simulink model "sampleModel119"  (R2021b)
settings: Solver=VariableStepAuto  StartTime=0.0  StopTime=10.0  RelTol=1e-3
undefined symbols (not defined in the file or in its folder): DiscIntNeverNeededParam, Newton, Raphson
libraries: simulink x14, slpidlib x1
settings Model: Creator=user  LastModifiedBy=user

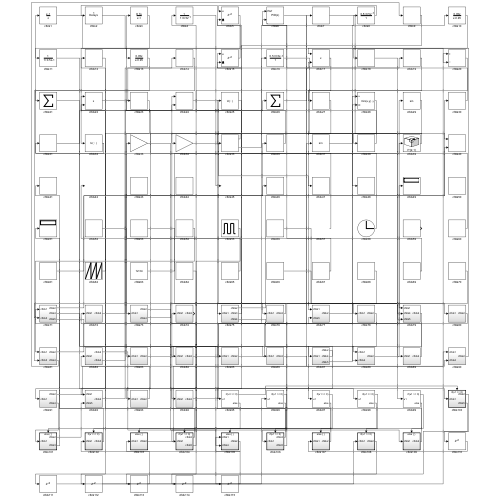
[thumbnail: Simulink's stored preview of the top-level diagram]
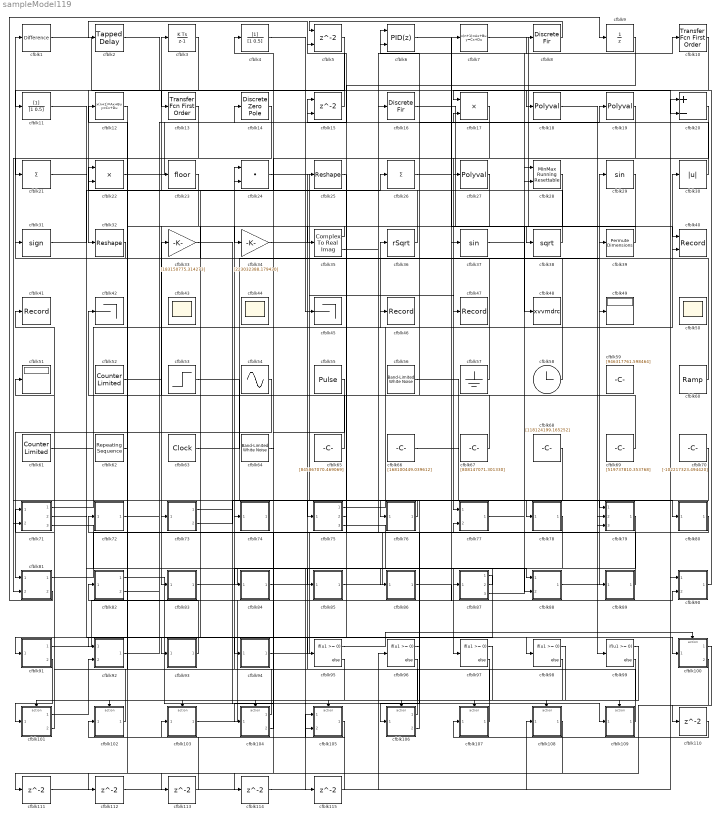
== system sampleModel119 ==
  cfblk1 : simulink/Discrete/Difference  ICPrevInput=0.0  OutMin=[]  OutMax=[]  OutDataTypeStr=Inherit: Inherit via back propagation  OutDataType=fixdt(1, 16)  OutScaling=2^-10  DoSatur=off
  cfblk10 : simulink/Discrete/Transfer Fcn First Order  PoleZ=0.95  ICPrevOutput=0.0  DoSatur=off
  cfblk100 : Subsystem  TreatAsAtomicUnit=on
  cfblk101 : Subsystem  TreatAsAtomicUnit=on
  cfblk102 : Subsystem  TreatAsAtomicUnit=on
  cfblk103 : Subsystem  TreatAsAtomicUnit=on
  cfblk104 : Subsystem  TreatAsAtomicUnit=on
  cfblk105 : Subsystem  TreatAsAtomicUnit=on
  cfblk106 : Subsystem  TreatAsAtomicUnit=on
  cfblk107 : Subsystem  TreatAsAtomicUnit=on
  cfblk108 : Subsystem  TreatAsAtomicUnit=on
  cfblk109 : Subsystem  TreatAsAtomicUnit=on
  cfblk11 : DiscreteFilter  SampleTime=1
  cfblk{110..115} (6 alike) : Delay  SampleTime=1
  cfblk12 : DiscreteStateSpace
  cfblk13 : simulink/Discrete/Transfer Fcn First Order  PoleZ=0.95  ICPrevOutput=0.0  DoSatur=off
  cfblk14 : DiscreteZeroPole  Poles=[0 0.5]  Gain=1
  cfblk15 : Delay  ShowEnablePort=on  SampleTime=1
      settings: InputPortMap=u0,e6
  cfblk16 : DiscreteFir  SampleTime=1
  cfblk17 : Product
  cfblk18 : Polyval  Coefs=[ +2.081618890e-019, -1.441693666e-014, +4.719686976e-010, -8.536869453e-006, +1.621573104e-001, -8.087801117e+001 ]
  cfblk19 : Polyval  Coefs=[ +2.081618890e-019, -1.441693666e-014, +4.719686976e-010, -8.536869453e-006, +1.621573104e-001, -8.087801117e+001 ]
  cfblk2 : simulink/Discrete/Tapped Delay  vinit=0.0  samptime=-1  NumDelays=1  DelayOrder=Oldest  includeCurrent=off
  cfblk20 : Sum  Inputs=+-
  cfblk21 : Sum  Inputs=+
  cfblk22 : Product  Inputs=**
  cfblk23 : Rounding
  cfblk24 : DotProduct  InputSameDT=on  OutDataTypeStr=Inherit: Inherit via internal rule
  cfblk25 : Reshape
  cfblk26 : Sum  Inputs=+
  cfblk27 : Polyval  Coefs=[ +2.081618890e-019, -1.441693666e-014, +4.719686976e-010, -8.536869453e-006, +1.621573104e-001, -8.087801117e+001 ]
  cfblk28 : simulink/Math Operations/MinMax Running Resettable  Function=min  vinit=0.0
  cfblk29 : Trigonometry
  cfblk3 : DiscreteIntegrator  ICPrevOutput=DiscIntNeverNeededParam  ICPrevScaledInput=DiscIntNeverNeededParam
  cfblk30 : Abs
  cfblk31 : Signum
  cfblk32 : Reshape
  cfblk33 : Gain  Gain=[183150775.314273]
  cfblk34 : Gain  Gain=[223032388.179430]
  cfblk35 : ComplexToRealImag
  cfblk36 : Sqrt  Operator=rSqrt  AlgorithmType=Newton-Raphson  SaturateOnIntegerOverflow=on
  cfblk37 : Trigonometry
  cfblk38 : Sqrt  SaturateOnIntegerOverflow=on
  cfblk39 : PermuteDimensions
  cfblk4 : DiscreteFilter  SampleTime=1
  cfblk40 : Record  FileSettingsInternal="{\"entries\":[{\"content\":{\"excelSettings\":{\"content\":{},\"type\":\"Streamout.ExcelSettings\"}},\"type\":\"Streamout.FileSettingStorage\",\"uuid\":\"4b90652c-f2d3-47f2-a44e-bcf3a3fec26d\"}],\"packageUris\":[\"http://schema.mathworks.com/mf0/streamout_blocks/R2020a\"],\"version\":\"1.0\"}"  Layout=[1 1]  SignalsInternal="{\"entries\":[{\"content\":{\"signals\":[{\"content\":{\"blockPath\":[\"sampleModel119/cfblk40\"],\"channel\":[],\"dimensions\":[1],\"domain\":\"sampleModel119/cfblk40\",\"lineColor\":\"#a2142f\",\"plots\":[1],\"port\":1,\"sid\":[\"\"],\"signalID\":4151,\"signalName\":\"cfblk6\"},\"type\":\"RecordBlkView.Signal\",\"uuid\":\"d5e0444b-39c8-4732-8124-8d2ee03c9154\"},{\"content\":{\"blockPath\":[\"sampleModel119/cfblk40\"],\"channel\":[],\"dimensions\":[1],\"domain\":\"sampleModel119/cfblk40\",\"lineColor\":\"#139fff\",\"plots\":[1],\"port\":2,\"sid\":[\"\"],\"signalID\":4155,\"signalName\":\"cfblk61\"},\"type\":\"RecordBlkView.Signal\",\"uuid\":\"776bc78c-e7e2-49e1-a7fd-18f1511b43d9\"}]},\"type\":\"RecordBlkView.InputSignals\",\"uuid\":\"2fea9de3-cc0b-4d57-9cd3-248ab124d388\"}],\"packageUris\":[\"http://schema.mathworks.com/mf0/streamout_blocks/R2020a\"],\"version\":\"1.0\"}"  VisualizationBindings="{\"xyplotplugin\":{\"info\":[{\"series\":[{\"bindingParametersList\":[{\"parameter\":\"X-Axis\",\"signalID\":4151,\"signalName\":\"cfblk6\"},{\"parameter\":\"Y-Axis\",\"signalID\":4155,\"signalName\":\"cfblk61\"}],\"seriesID\":3220}],\"subplotID\":1}]}}"  CompatibilityTag=XY
  cfblk41 : Record  FileSettingsInternal="{\"entries\":[{\"content\":{\"excelSettings\":{\"content\":{},\"type\":\"Streamout.ExcelSettings\"}},\"type\":\"Streamout.FileSettingStorage\",\"uuid\":\"8c36c4d4-0469-459e-8325-57697a053134\"}],\"packageUris\":[\"http://schema.mathworks.com/mf0/streamout_blocks/R2020a\"],\"version\":\"1.0\"}"  SignalsInternal="{\"entries\":[{\"content\":{\"signals\":[{\"content\":{\"blockPath\":[\"sampleModel119/cfblk41\"],\"channel\":[],\"dimensions\":[1],\"domain\":\"sampleModel119/cfblk41\",\"lineColor\":\"#fe330a\",\"plots\":[1],\"port\":1,\"sid\":[\"\"],\"signalID\":4159,\"signalName\":\"cfblk104:1\"},\"type\":\"RecordBlkView.Signal\",\"uuid\":\"6d2d44fb-15cd-4da0-8e52-60f91c5e197b\"}]},\"type\":\"RecordBlkView.InputSignals\",\"uuid\":\"76cdbd26-62aa-4d26-a689-d7fa7566e8ef\"}],\"packageUris\":[\"http://schema.mathworks.com/mf0/streamout_blocks/R2020a\"],\"version\":\"1.0\"}"  VisualizationBindings="{\"sparklinesplugin\":{\"info\":[{\"bindingParametersList\":[],\"subplotID\":1}]}}"
  cfblk42 : Terminator
  cfblk43 : Scope
      settings: Floating=on
  cfblk44 : Scope
      settings: Floating=on
  cfblk45 : Terminator
  cfblk46 : Record  FileSettingsInternal="{\"entries\":[{\"content\":{\"excelSettings\":{\"content\":{},\"type\":\"Streamout.ExcelSettings\"}},\"type\":\"Streamout.FileSettingStorage\",\"uuid\":\"35d2fa41-f68c-4e08-ac86-24c0cc6052f6\"}],\"packageUris\":[\"http://schema.mathworks.com/mf0/streamout_blocks/R2020a\"],\"version\":\"1.0\"}"  SignalsInternal="{\"entries\":[{\"content\":{\"signals\":[{\"content\":{\"blockPath\":[\"sampleModel119/cfblk46\"],\"channel\":[],\"dimensions\":[1],\"domain\":\"sampleModel119/cfblk46\",\"lineColor\":\"#22b573\",\"plots\":[1],\"port\":1,\"sid\":[\"\"],\"signalID\":4163,\"signalName\":\"cfblk72\"},\"type\":\"RecordBlkView.Signal\",\"uuid\":\"6c816a1f-c12f-4d80-813e-4e8bf75e3cfa\"}]},\"type\":\"RecordBlkView.InputSignals\",\"uuid\":\"aab32150-6d44-4daa-b8cf-e47eaa1a11c6\"}],\"packageUris\":[\"http://schema.mathworks.com/mf0/streamout_blocks/R2020a\"],\"version\":\"1.0\"}"  VisualizationBindings="{\"sparklinesplugin\":{\"info\":[{\"bindingParametersList\":[],\"subplotID\":1}]}}"
  cfblk47 : Record  FileSettingsInternal="{\"entries\":[{\"content\":{\"excelSettings\":{\"content\":{},\"type\":\"Streamout.ExcelSettings\"}},\"type\":\"Streamout.FileSettingStorage\",\"uuid\":\"1cc15422-dbef-4f88-bbe8-034119ca05b7\"}],\"packageUris\":[\"http://schema.mathworks.com/mf0/streamout_blocks/R2020a\"],\"version\":\"1.0\"}"  SignalsInternal="{\"entries\":[{\"content\":{\"signals\":[{\"content\":{\"blockPath\":[\"sampleModel119/cfblk47\"],\"channel\":[],\"dimensions\":[1,1],\"domain\":\"sampleModel119/cfblk47\",\"lineColor\":\"#0072bd\",\"plots\":[1],\"port\":1,\"sid\":[\"\"],\"signalID\":4167,\"signalName\":\"cfblk34\"},\"type\":\"RecordBlkView.Signal\",\"uuid\":\"1ed8d035-bae1-4148-97b8-32f6098d1f51\"}]},\"type\":\"RecordBlkView.InputSignals\",\"uuid\":\"92e54281-6170-43a9-afc8-92f9430844b9\"}],\"packageUris\":[\"http://schema.mathworks.com/mf0/streamout_blocks/R2020a\"],\"version\":\"1.0\"}"  VisualizationBindings="{\"sparklinesplugin\":{\"info\":[{\"bindingParametersList\":[],\"subplotID\":1}]}}"
  cfblk48 : ToWorkspace  VariableName=xvvmdrc  SaveFormat=Timeseries  SampleTime=-1
  cfblk49 : Display
  cfblk5 : Delay  ShowEnablePort=on  SampleTime=1
      settings: InputPortMap=u0,e6
  cfblk50 : Scope
      settings: Floating=on
  cfblk51 : Display
  cfblk52 : simulink/Sources/Counter Limited  uplimit=[61.000000]  tsamp=-1
  cfblk53 : Step  Time=[34.000000]  Before=[46179549.003824]  After=[835001809.897906]  SampleTime=0
  cfblk54 : Sin  Amplitude=[-89702734.800295]  Bias=[573127760.762597]  SampleTime=0
  cfblk55 : DiscretePulseGenerator  PulseType=Time based  Amplitude=[-241727286.164151]  Period=[40925784.883433]  PulseWidth=5  PhaseDelay=[9.000000]
  cfblk56 : simulink/Sources/Band-Limited White Noise  Cov=[2484773712.290704]  Ts=0.1  seed=[484627539.000000]
  cfblk57 : Ground
  cfblk58 : Clock
  cfblk59 : Constant  Value=[946317761.598464]  SampleTime=1
  cfblk6 : slpidlib/PID Controller (2DOF)  Controller=PID  Form=Parallel  TimeDomain=Discrete-time  UseExternalTs=off  SampleTime=1  IntegratorMethod=Forward Euler  FilterMethod=Forward Euler  ControllerParametersSource=internal  P=1  I=1  D=0  UseFilter=on  N=100  b=1  c=1  TunerSelectOption=Transfer Function Based (PID Tuner App)  InitialConditionSource=internal  InitialConditionForIntegrator=0  InitialConditionForFilter=0  DifferentiatorICPrevScaledInput=0  ExternalReset=none  TrackingMode=off  Kt=1  LimitOutput=off  SatLimitsSource=internal  UpperSaturationLimit=inf  LowerSaturationLimit=-inf  LinearizeAsGain=off  AntiWindupMode=none  Kb=1  POutMin=[]  POutMax=[]  IOutMin=[]  IOutMax=[]  DOutMin=[]  DOutMax=[]  NOutMin=[]  NOutMax=[]  bOutMin=[]  bOutMax=[]  cOutMin=[]  cOutMax=[]  SumOutMin=[]  SumOutMax=[]  SaturationOutMin=[]  SaturationOutMax=[]  PParamMin=[]  PParamMax=[]  IParamMin=[]  IParamMax=[]  DParamMin=[]  DParamMax=[]  NParamMin=[]  NParamMax=[]  bParamMin=[]  bParamMax=[]  cParamMin=[]  cParamMax=[]  KbParamMin=[]  KbParamMax=[]  KtParamMin=[]  KtParamMax=[]  KbOutMin=[]  KbOutMax=[]  KtOutMin=[]  KtOutMax=[]  IntegratorOutMin=[]  IntegratorOutMax=[]  FilterOutMin=[]  FilterOutMax=[]  SumI1OutMin=[]  SumI1OutMax=[]  SumI2OutMin=[]  SumI2OutMax=[]  SumI3OutMin=[]  SumI3OutMax=[]  SumI4OutMin=[]  SumI4OutMax=[]  SumDOutMin=[]  SumDOutMax=[]  Sum1OutMin=[]  Sum1OutMax=[]  Sum2OutMin=[]  Sum2OutMax=[]  Sum3OutMin=[]  Sum3OutMax=[]  DifferentiatorOutMin=[]  DifferentiatorOutMax=[]  FilterDiffOutCoefMin=[]  FilterDiffOutCoefMax=[]  ReciprocalOutMin=[]  ReciprocalOutMax=[]  SumDenOutMin=[]  SumDenOutMax=[]  SumNumOutMin=[]  SumNumOutMax=[]  DivideOutMin=[]  DivideOutMax=[]  UdiffTsProdOutMin=[]  UdiffTsProdOutMax=[]  NTsProdOutMin=[]  NTsProdOutMax=[]  UintegralTsProdOutMin=[]  UintegralTsProdOutMax=[]  UngainTsProdOutMin=[]  UngainTsProdOutMax=[]  IntegratorContinuousStateAttributes=''  IntegratorStateMustResolveToSignalObject=off  IntegratorRTWStateStorageClass=Auto  FilterContinuousStateAttributes=''  FilterStateMustResolveToSignalObject=off  FilterRTWStateStorageClass=Auto  ParallelPVariant=InternalParameters  IdealPVariant=Disabled  IVariant=InternalParameters  DVariant=InternalParameters  bVariant=InternalParameters  cVariant=InternalParameters  IntegratorVariant=Discrete  SatVariant=Disabled  AWVariant=Passthrough  PCopyVariant=Disabled  TRVariant=Disabled  FdbkBlocksVariant=Forward  IdealPFdbkVariant=Disabled  SatFdbkVariant=Disabled  DerivativeFilterVariant=ForwardEulerFilter  NVariant=InternalParameters  NCopyVariant=Disabled  FilterICVariant=InternalICsFilter  IntegratorICVariant=InternalICs  ExternalResetVariant=Disabled  TRSumVariant=Passthrough  SumFdbkVariant=Disabled  SumVariant=Sum_PID  TsampFilterVariant=InternalTs  TsampNgainVariant=Passthrough  TsampIntegralVariant=Passthrough  ExternalSaturationOutDataTypeStr=Inherit: Same as second input
      settings: SourceProductBaseCode=SL
  cfblk60 : simulink/Sources/Ramp  slope=[5825.161716]  start=[33.046930]  InitialOutput=[-744615.276232]
  cfblk61 : simulink/Sources/Counter Limited  uplimit=[442.000000]  tsamp=-1
  cfblk62 : simulink/Sources/Repeating Sequence  rep_seq_t=[0 2]  rep_seq_y=[-993841258.890816, 268026566.571388]
  cfblk63 : DigitalClock
  cfblk64 : simulink/Sources/Band-Limited White Noise  Cov=[6507311425.437892]  Ts=0.1  seed=[1699256714.000000]
  cfblk65 : Constant  Value=[845867070.469069]  SampleTime=1
  cfblk66 : Constant  Value=[168100449.039612]  SampleTime=1
  cfblk67 : Constant  Value=[808147071.301330]  SampleTime=1
  cfblk68 : Constant  Value=[118124199.165252]  SampleTime=1
  cfblk69 : Constant  Value=[519737810.353768]  SampleTime=1
  cfblk7 : DiscreteStateSpace
  cfblk70 : Constant  Value=[-102217323.494420]  SampleTime=1
  cfblk71 : Subsystem
  cfblk72 : Subsystem
  cfblk73 : Subsystem
  cfblk74 : Subsystem
  cfblk75 : Subsystem
  cfblk76 : Subsystem
  cfblk77 : Subsystem
  cfblk78 : Subsystem
  cfblk79 : Subsystem
  cfblk8 : DiscreteFir  SampleTime=1
  cfblk80 : Subsystem
  cfblk81 : Subsystem
  cfblk82 : Subsystem
  cfblk83 : Subsystem
  cfblk84 : Subsystem
  cfblk85 : Subsystem
  cfblk86 : Subsystem
  cfblk87 : Subsystem
  cfblk88 : Subsystem
  cfblk89 : Subsystem
  cfblk9 : UnitDelay  HasFrameUpgradeWarning=on
  cfblk90 : Subsystem
  cfblk91 : Subsystem
  cfblk92 : Subsystem
  cfblk93 : Subsystem
  cfblk94 : Subsystem
  cfblk{95..99} (5 alike) : If  IfExpression=u1 >= 0  SampleTime=1
  wires:
  cfblk93/1(cfblk2) -> cfblk82/1(cfblk1)
  cfblk3/1 -> cfblk32/1
  cfblk63/1 -> cfblk29/1
  cfblk81/1(cfblk2) -> cfblk39/1
  cfblk106/1(cfblk2) -> cfblk24/1
  cfblk105/1(cfblk2) -> cfblk102/1(cfblk1)
  cfblk19/1 -> cfblk77/1(cfblk1)
  cfblk78/1(cfblk2) -> cfblk97/1
  cfblk38/1 -> cfblk3/1
  cfblk53/1 -> cfblk76/1(cfblk1)
  cfblk24/1 -> cfblk78/1(cfblk1)
  cfblk1/1 -> cfblk13/1
  cfblk32/1 -> cfblk1/1
  cfblk91/1(cfblk2) -> cfblk37/1
  cfblk80/1(cfblk2) -> cfblk77/2(cfblk5)
  cfblk83/1(cfblk2) -> cfblk87/1(cfblk1)
  cfblk109/1(cfblk2) -> cfblk25/1
  cfblk29/1 -> cfblk38/1
  cfblk76/1(cfblk2) -> cfblk75/1(cfblk1)
  cfblk107/1(cfblk2) -> cfblk12/1
  cfblk82/1(cfblk2) -> cfblk109/1(cfblk1)
  cfblk75/1(cfblk2) -> cfblk30/1
  cfblk87/1(cfblk2) -> cfblk91/1(cfblk1)
  cfblk16/1 -> cfblk48/1
  cfblk62/1 -> cfblk22/1
  cfblk66/1 -> cfblk80/1(cfblk1)
  cfblk87/2(cfblk4) -> cfblk84/1(cfblk1)
  cfblk106/2(cfblk5) -> cfblk72/1(cfblk1)
  cfblk90/1(cfblk2) -> cfblk17/1
  cfblk35/1 -> cfblk34/1
  cfblk71/1(cfblk2) -> cfblk36/1
  cfblk4/1 -> cfblk45/1
  cfblk54/1 -> cfblk81/1(cfblk1)
  cfblk103/1(cfblk2) -> cfblk20/1
  cfblk15/1 -> cfblk2/1
  cfblk88/1(cfblk2) -> cfblk49/1
  cfblk9/1 -> cfblk15/1
  cfblk22/1 -> cfblk17/2
  cfblk60/1 -> cfblk31/1
  cfblk84/1(cfblk2) -> cfblk7/1
  cfblk34/1 -> cfblk47/1
  cfblk52/1 -> cfblk83/1(cfblk1)
  cfblk7/1 -> cfblk89/1(cfblk1)
  cfblk94/1(cfblk2) -> cfblk16/1
  cfblk23/1 -> cfblk73/1(cfblk1)
  cfblk102/1(cfblk2) -> cfblk71/1(cfblk1)
  cfblk2/1 -> cfblk20/2
  cfblk6/1 -> cfblk40/1
  cfblk68/1 -> cfblk71/2(cfblk3)
  cfblk87/3(cfblk5) -> cfblk28/1
  cfblk64/1 -> cfblk94/1(cfblk1)
  cfblk14/1 -> cfblk21/1
  cfblk30/1 -> cfblk6/1
  cfblk67/1 -> cfblk33/1
  cfblk70/1 -> cfblk106/1(cfblk1)
  cfblk104/1(cfblk2) -> cfblk41/1
  cfblk55/1 -> cfblk104/1(cfblk1)
  cfblk58/1 -> cfblk23/1
  cfblk104/2(cfblk5) -> cfblk74/1(cfblk1)
  cfblk85/1(cfblk2) -> cfblk28/2
  cfblk65/1 -> cfblk42/1
  cfblk39/1 -> cfblk35/1
  cfblk35/2 -> cfblk8/1
  cfblk20/1 -> cfblk27/1
  cfblk31/1 -> cfblk24/2
  cfblk73/1(cfblk2) -> cfblk100/1(cfblk1)
  cfblk8/1 -> cfblk5/1
  cfblk91/2(cfblk4) -> cfblk101/1(cfblk1)
  cfblk57/1 -> cfblk5/2
  cfblk72/1(cfblk2) -> cfblk46/1
  cfblk82/2(cfblk4) -> cfblk14/1
  cfblk71/2(cfblk4) -> cfblk85/1(cfblk1)
  cfblk37/1 -> cfblk10/1
  cfblk75/2(cfblk3) -> cfblk22/2
  cfblk56/1 -> cfblk99/1
  cfblk13/1 -> cfblk81/2(cfblk3)
  cfblk33/1 -> cfblk105/2(cfblk4)
  cfblk36/1 -> cfblk4/1
  cfblk12/1 -> cfblk92/1(cfblk1)
  cfblk25/1 -> cfblk95/1
  cfblk10/1 -> cfblk18/1
  cfblk21/1 -> cfblk86/1(cfblk1)
  cfblk75/3(cfblk4) -> cfblk88/1(cfblk1)
  cfblk73/2(cfblk4) -> cfblk79/1(cfblk1)
  cfblk61/1 -> cfblk40/2
  cfblk5/1 -> cfblk11/1
  cfblk28/1 -> cfblk93/1(cfblk1)
  cfblk89/1(cfblk2) -> cfblk15/2
  cfblk81/2(cfblk4) -> cfblk9/1
  cfblk11/1 -> cfblk98/1
  cfblk77/1(cfblk2) -> cfblk79/2(cfblk4)
  cfblk79/1(cfblk2) -> cfblk88/2(cfblk4)
  cfblk101/1(cfblk2) -> cfblk92/2(cfblk5)
  cfblk101/2(cfblk3) -> cfblk51/1
  cfblk18/1 -> cfblk79/3(cfblk5)
  cfblk69/1 -> cfblk6/2
  cfblk26/1 -> cfblk19/1
  cfblk86/1(cfblk2) -> cfblk90/2(cfblk4)
  cfblk92/1(cfblk2) -> cfblk26/1
  cfblk95/1 -> cfblk100/Action
  cfblk95/2 -> cfblk101/Action
  cfblk96/1 -> cfblk102/Action
  cfblk96/2 -> cfblk103/Action
  cfblk97/1 -> cfblk104/Action
  cfblk97/2 -> cfblk105/Action
  cfblk98/1 -> cfblk106/Action
  cfblk98/2 -> cfblk107/Action
  cfblk99/1 -> cfblk108/Action
  cfblk99/2 -> cfblk109/Action
  cfblk100/1(cfblk2) -> cfblk110/1
  cfblk110/1 -> cfblk107/1(cfblk1)
  cfblk100/2(cfblk5) -> cfblk111/1
  cfblk111/1 -> cfblk96/1
  cfblk27/1 -> cfblk112/1
  cfblk112/1 -> cfblk108/1(cfblk1)
  cfblk108/1(cfblk2) -> cfblk113/1
  cfblk113/1 -> cfblk103/1(cfblk1)
  cfblk17/1 -> cfblk114/1
  cfblk114/1 -> cfblk90/1(cfblk1)
  cfblk71/3(cfblk5) -> cfblk115/1
  cfblk115/1 -> cfblk105/1(cfblk1)

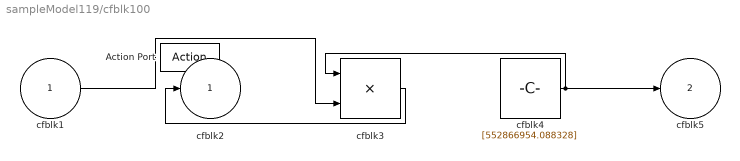
== system sampleModel119/cfblk100 ==
  cfblk1 : Inport
  Action Port : ActionPort  ActionPortLabel=if(u1 >= 0)
  cfblk3 : Product  Inputs=**
  cfblk4 : Constant  Value=[552866954.088328]  SampleTime=1
  cfblk2 : Outport
  cfblk5 : Outport  Port=2
  wires:
  cfblk4/1 -> cfblk3/1, cfblk5/1
  cfblk3/1 -> cfblk2/1
  cfblk1/1 -> cfblk3/2

== system sampleModel119/cfblk101 ==
  cfblk1 : Inport
  Action Port : ActionPort  ActionPortLabel=else
  cfblk2 : Outport
  cfblk3 : Outport  Port=2
  wires:
  cfblk1/1 -> cfblk3/1, cfblk2/1

== system sampleModel119/cfblk102 ==
  cfblk1 : Inport
  Action Port : ActionPort  ActionPortLabel=if(u1 >= 0)
  cfblk3 : simulink/Discrete/Transfer Fcn Real Zero  ZeroZ=0.75  ICPrevInput=0.0  DoSatur=off
      settings: SourceProductBaseCode=SL
  cfblk2 : Outport
  wires:
  cfblk3/1 -> cfblk2/1
  cfblk1/1 -> cfblk3/1

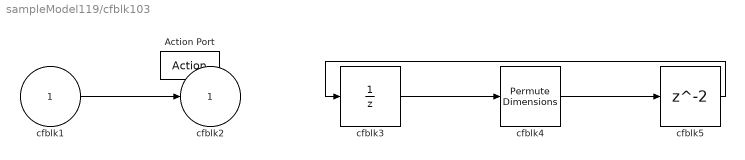
== system sampleModel119/cfblk103 ==
  cfblk1 : Inport
  Action Port : ActionPort  ActionPortLabel=else
  cfblk3 : UnitDelay  SampleTime=-1  HasFrameUpgradeWarning=on
  cfblk4 : PermuteDimensions
  cfblk5 : Delay
  cfblk2 : Outport
  wires:
  cfblk1/1 -> cfblk2/1
  cfblk3/1 -> cfblk4/1
  cfblk4/1 -> cfblk5/1
  cfblk5/1 -> cfblk3/1

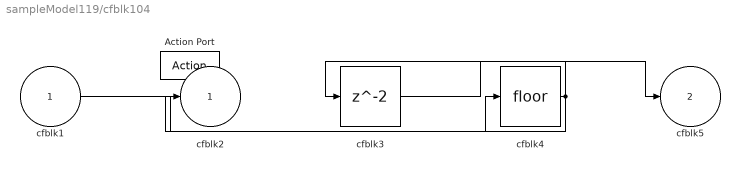
== system sampleModel119/cfblk104 ==
  cfblk1 : Inport
  Action Port : ActionPort  ActionPortLabel=if(u1 >= 0)
  cfblk3 : Delay
  cfblk4 : Rounding
  cfblk2 : Outport
  cfblk5 : Outport  Port=2
  wires:
  cfblk1/1 -> cfblk4/1
  cfblk4/1 -> cfblk3/1, cfblk2/1
  cfblk3/1 -> cfblk5/1

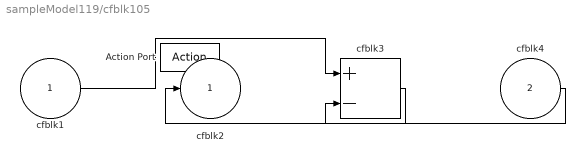
== system sampleModel119/cfblk105 ==
  cfblk1 : Inport
  cfblk4 : Inport  Port=2
  Action Port : ActionPort  ActionPortLabel=else
  cfblk3 : Sum  Inputs=+-
  cfblk2 : Outport
  wires:
  cfblk3/1 -> cfblk2/1
  cfblk1/1 -> cfblk3/1
  cfblk4/1 -> cfblk3/2

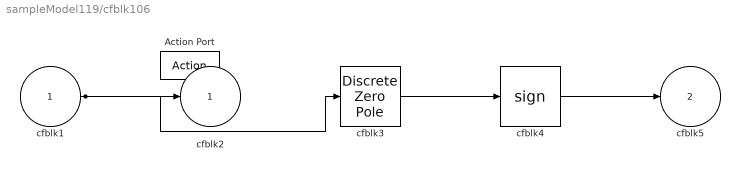
== system sampleModel119/cfblk106 ==
  cfblk1 : Inport
  Action Port : ActionPort  ActionPortLabel=if(u1 >= 0)
  cfblk3 : DiscreteZeroPole  Poles=[0 0.5]  Gain=1  SampleTime=-1
  cfblk4 : Signum
  cfblk2 : Outport
  cfblk5 : Outport  Port=2
  wires:
  cfblk1/1 -> cfblk2/1, cfblk3/1
  cfblk3/1 -> cfblk4/1
  cfblk4/1 -> cfblk5/1

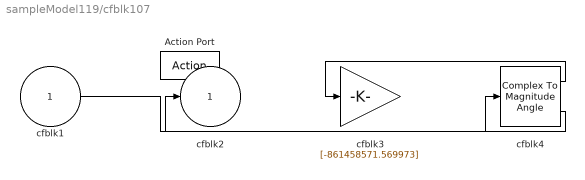
== system sampleModel119/cfblk107 ==
  cfblk1 : Inport
  Action Port : ActionPort  ActionPortLabel=else
  cfblk3 : Gain  Gain=[-861458571.569973]
  cfblk4 : ComplexToMagnitudeAngle
  cfblk2 : Outport
  wires:
  cfblk4/1 -> cfblk3/1
  cfblk4/2 -> cfblk2/1
  cfblk1/1 -> cfblk4/1

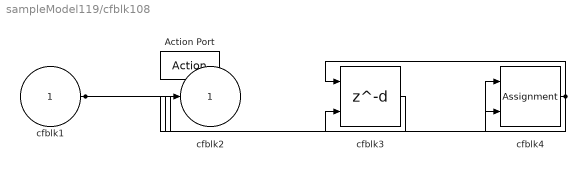
== system sampleModel119/cfblk108 ==
  cfblk1 : Inport
  Action Port : ActionPort  ActionPortLabel=if(u1 >= 0)
  cfblk3 : Delay  DelayLengthSource=Input port
      settings: InputPortMap=u0,p1
  cfblk4 : Assignment  DiagnosticForDimensions=Warning  IndexOptions=Index vector (dialog)  Indices=1  OutputSizes=1
  cfblk2 : Outport
  wires:
  cfblk4/1 -> cfblk3/1, cfblk3/2
  cfblk1/1 -> cfblk4/1, cfblk4/2
  cfblk3/1 -> cfblk2/1

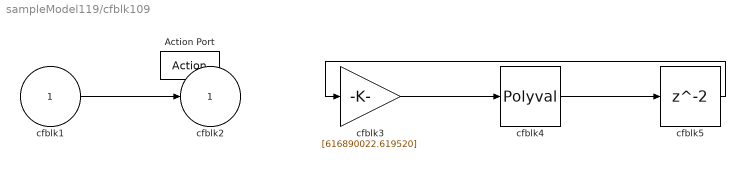
== system sampleModel119/cfblk109 ==
  cfblk1 : Inport
  Action Port : ActionPort  ActionPortLabel=else
  cfblk3 : Gain  Gain=[616890022.619520]
  cfblk4 : Polyval  Coefs=[ +2.081618890e-019, -1.441693666e-014, +4.719686976e-010, -8.536869453e-006, +1.621573104e-001, -8.087801117e+001 ]
  cfblk5 : Delay
  cfblk2 : Outport
  wires:
  cfblk1/1 -> cfblk2/1
  cfblk3/1 -> cfblk4/1
  cfblk4/1 -> cfblk5/1
  cfblk5/1 -> cfblk3/1

== system sampleModel119/cfblk71 ==
  cfblk1 : Inport
  cfblk3 : Inport  Port=2
  cfblk2 : Outport
  cfblk4 : Outport  Port=2
  cfblk5 : Outport  Port=3
  wires:
  cfblk3/1 -> cfblk2/1
  cfblk1/1 -> cfblk4/1, cfblk5/1

== system sampleModel119/cfblk72 ==
  cfblk1 : Inport
  cfblk3 : DiscreteIntegrator  ICPrevOutput=DiscIntNeverNeededParam  ICPrevScaledInput=DiscIntNeverNeededParam
  cfblk4 : Product  Inputs=*
  cfblk2 : Outport
  wires:
  cfblk1/1 -> cfblk3/1
  cfblk3/1 -> cfblk4/1
  cfblk4/1 -> cfblk2/1

== system sampleModel119/cfblk73 ==
  cfblk1 : Inport
  cfblk3 : Sqrt  SaturateOnIntegerOverflow=on
  cfblk2 : Outport
  cfblk4 : Outport  Port=2
  wires:
  cfblk3/1 -> cfblk4/1
  cfblk1/1 -> cfblk2/1, cfblk3/1

== system sampleModel119/cfblk74 ==
  cfblk1 : Inport
  cfblk3 : Trigonometry
  cfblk2 : Outport
  wires:
  cfblk1/1 -> cfblk2/1, cfblk3/1

== system sampleModel119/cfblk75 ==
  cfblk1 : Inport
  cfblk2 : Outport
  cfblk3 : Outport  Port=2
  cfblk4 : Outport  Port=3
  wires:
  cfblk1/1 -> cfblk4/1, cfblk3/1, cfblk2/1

== system sampleModel119/cfblk76 ==
  cfblk1 : Inport
  cfblk3 : DiscreteTransferFcn  SampleTime=1
  cfblk2 : Outport
  wires:
  cfblk1/1 -> cfblk2/1, cfblk3/1

== system sampleModel119/cfblk77 ==
  cfblk1 : Inport
  cfblk5 : Inport  Port=2
  cfblk3 : simulink/Discrete/Transfer Fcn Real Zero  ZeroZ=0.75  ICPrevInput=0.0  DoSatur=off
      settings: SourceProductBaseCode=SL
  cfblk4 : Rounding
  cfblk2 : Outport
  wires:
  cfblk5/1 -> cfblk3/1
  cfblk4/1 -> cfblk2/1
  cfblk3/1 -> cfblk4/1

== system sampleModel119/cfblk78 ==
  cfblk1 : Inport
  cfblk3 : Sin  TimeSource=Use external signal  SampleTime=0
  cfblk2 : Outport
  wires:
  cfblk1/1 -> cfblk2/1, cfblk3/1

== system sampleModel119/cfblk79 ==
  cfblk1 : Inport
  cfblk4 : Inport  Port=2
  cfblk5 : Inport  Port=3
  cfblk3 : Constant  Value=[407942540.240208]  SampleTime=1
  cfblk2 : Outport
  wires:
  cfblk1/1 -> cfblk2/1

== system sampleModel119/cfblk80 ==
  cfblk1 : Inport
  cfblk3 : UnaryMinus
  cfblk4 : Polyval  Coefs=[ +2.081618890e-019, -1.441693666e-014, +4.719686976e-010, -8.536869453e-006, +1.621573104e-001, -8.087801117e+001 ]
  cfblk2 : Outport
  wires:
  cfblk3/1 -> cfblk2/1
  cfblk1/1 -> cfblk4/1
  cfblk4/1 -> cfblk3/1

== system sampleModel119/cfblk81 ==
  cfblk1 : Inport
  cfblk3 : Inport  Port=2
  cfblk2 : Outport
  cfblk4 : Outport  Port=2
  wires:
  cfblk3/1 -> cfblk2/1
  cfblk1/1 -> cfblk4/1

== system sampleModel119/cfblk82 ==
  cfblk1 : Inport
  cfblk3 : UnaryMinus
  cfblk2 : Outport
  cfblk4 : Outport  Port=2
  wires:
  cfblk1/1 -> cfblk4/1, cfblk3/1
  cfblk3/1 -> cfblk2/1

== system sampleModel119/cfblk83 ==
  cfblk1 : Inport
  cfblk3 : Product  Inputs=**
  cfblk2 : Outport
  wires:
  cfblk1/1 -> cfblk3/1, cfblk3/2
  cfblk3/1 -> cfblk2/1

== system sampleModel119/cfblk84 ==
  cfblk1 : Inport
  cfblk3 : DiscreteIntegrator  ICPrevOutput=DiscIntNeverNeededParam  ICPrevScaledInput=DiscIntNeverNeededParam
  cfblk2 : Outport
  wires:
  cfblk1/1 -> cfblk3/1
  cfblk3/1 -> cfblk2/1

== system sampleModel119/cfblk85 ==
  cfblk1 : Inport
  cfblk3 : simulink/Discrete/Tapped Delay  vinit=0.0  samptime=-1  NumDelays=1  DelayOrder=Oldest  includeCurrent=off
  cfblk2 : Outport
  wires:
  cfblk1/1 -> cfblk2/1, cfblk3/1

== system sampleModel119/cfblk86 ==
  cfblk1 : Inport
  cfblk3 : Assignment  DiagnosticForDimensions=Warning  IndexOptions=Index vector (dialog)  Indices=1  OutputSizes=1
  cfblk4 : Sum  Inputs=+
  cfblk5 : Delay  SampleTime=1
  cfblk2 : Outport
  wires:
  cfblk4/1 -> cfblk2/1, cfblk5/1
  cfblk3/1 -> cfblk4/1
  cfblk1/1 -> cfblk3/2
  cfblk5/1 -> cfblk3/1

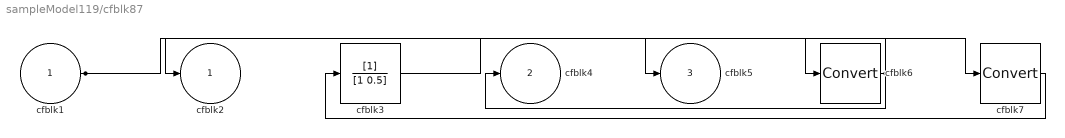
== system sampleModel119/cfblk87 ==
  cfblk1 : Inport
  cfblk3 : DiscreteFilter  SampleTime=1
  cfblk6 : DataTypeConversion
  cfblk7 : DataTypeConversion
  cfblk2 : Outport
  cfblk4 : Outport  Port=2
  cfblk5 : Outport  Port=3
  wires:
  cfblk1/1 -> cfblk5/1, cfblk7/1
  cfblk3/1 -> cfblk6/1
  cfblk6/1 -> cfblk4/1, cfblk2/1
  cfblk7/1 -> cfblk3/1

== system sampleModel119/cfblk88 ==
  cfblk1 : Inport
  cfblk4 : Inport  Port=2
  cfblk3 : Sqrt  SaturateOnIntegerOverflow=on
  cfblk2 : Outport
  wires:
  cfblk1/1 -> cfblk3/1
  cfblk3/1 -> cfblk2/1

== system sampleModel119/cfblk89 ==
  cfblk1 : Inport
  cfblk3 : DiscreteFir  SampleTime=1
  cfblk4 : Delay  DelayLengthSource=Input port  SampleTime=1
      settings: InputPortMap=u0,p1
  cfblk5 : Constant  Value=[-877351926.643604]  SampleTime=1
  cfblk2 : Outport
  wires:
  cfblk1/1 -> cfblk2/1
  cfblk3/1 -> cfblk4/1, cfblk4/2
  cfblk5/1 -> cfblk3/1

== system sampleModel119/cfblk90 ==
  cfblk1 : Inport
  cfblk4 : Inport  Port=2
  cfblk3 : Squeeze
  cfblk2 : Outport
  wires:
  cfblk1/1 -> cfblk2/1
  cfblk4/1 -> cfblk3/1

== system sampleModel119/cfblk91 ==
  cfblk1 : Inport
  cfblk3 : Assignment  DiagnosticForDimensions=Warning  IndexOptions=Index vector (dialog)  Indices=1  OutputSizes=1
  cfblk2 : Outport
  cfblk4 : Outport  Port=2
  wires:
  cfblk3/1 -> cfblk2/1
  cfblk1/1 -> cfblk4/1, cfblk3/1, cfblk3/2

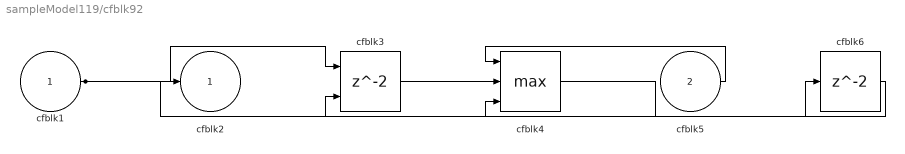
== system sampleModel119/cfblk92 ==
  cfblk1 : Inport
  cfblk5 : Inport  Port=2
  cfblk3 : Delay  ShowEnablePort=on  SampleTime=1
      settings: InputPortMap=u0,e6
  cfblk4 : MinMax  Function=max  Inputs=3
  cfblk6 : Delay  SampleTime=1
  cfblk2 : Outport
  wires:
  cfblk5/1 -> cfblk4/1
  cfblk1/1 -> cfblk3/1, cfblk2/1, cfblk4/3
  cfblk3/1 -> cfblk4/2
  cfblk4/1 -> cfblk6/1
  cfblk6/1 -> cfblk3/2

== system sampleModel119/cfblk93 ==
  cfblk1 : Inport
  cfblk3 : DiscreteStateSpace
  cfblk4 : DataTypeConversion
  cfblk2 : Outport
  wires:
  cfblk3/1 -> cfblk2/1
  cfblk1/1 -> cfblk4/1
  cfblk4/1 -> cfblk3/1

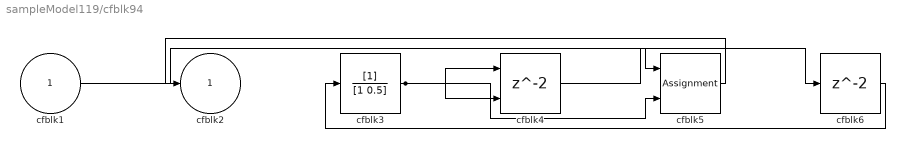
== system sampleModel119/cfblk94 ==
  cfblk1 : Inport
  cfblk3 : DiscreteFilter  SampleTime=1
  cfblk4 : Delay  ShowEnablePort=on  SampleTime=1
      settings: InputPortMap=u0,e6
  cfblk5 : Assignment  DiagnosticForDimensions=Warning  IndexOptions=Index vector (dialog)  Indices=1  OutputSizes=1
  cfblk6 : Delay  SampleTime=1
  cfblk2 : Outport
  wires:
  cfblk1/1 -> cfblk5/1
  cfblk5/1 -> cfblk2/1
  cfblk3/1 -> cfblk5/2, cfblk4/1, cfblk4/2
  cfblk4/1 -> cfblk6/1
  cfblk6/1 -> cfblk3/1
